simulink model "tutorial36_stateflow"  (R2025a)
settings: Solver=VariableStepAuto  StartTime=0.0  StopTime=10.0  RelTol=1e-3
settings Model: Creator=xing2  LastModifiedBy=xing2

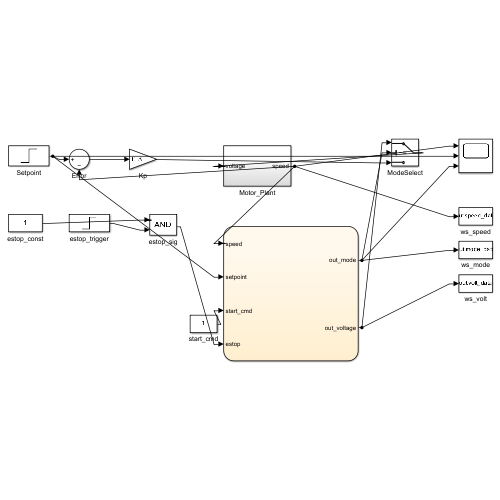
[thumbnail: Simulink's stored preview of the top-level diagram]
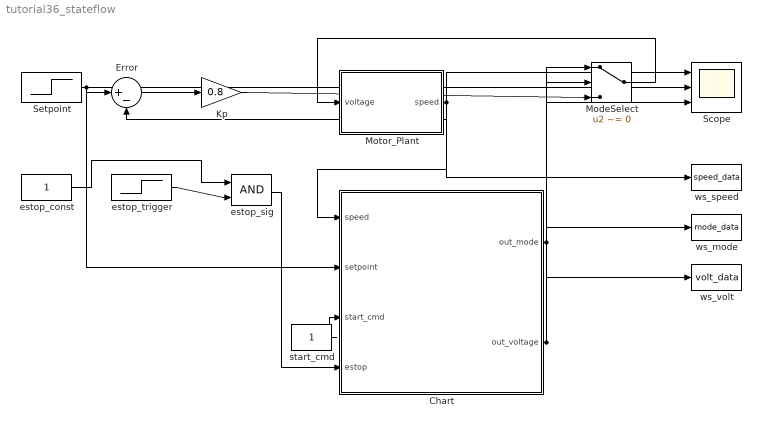
== system tutorial36_stateflow ==
  Chart : Stateflow chart  TreatAsAtomicUnit=on
  Error : Sum  Inputs=|+-
  Kp : Gain  Gain=0.8
  ModeSelect : Switch  Criteria=u2 ~= 0  SaturateOnIntegerOverflow=off  InputSameDT=off
  Motor_Plant : Subsystem
  Scope : Scope  NumInputPorts=3
  Setpoint : Step  Time=0.5  After=100  SampleTime=0
  estop_const : Constant
  estop_sig : Logic  AllPortsSameDT=off  OutDataTypeStr=boolean
  estop_trigger : Step  Time=8  SampleTime=0
  start_cmd : Constant
  ws_mode : ToWorkspace  VariableName=mode_data  SaveFormat=Timeseries  SampleTime=-1
  ws_speed : ToWorkspace  VariableName=speed_data  SaveFormat=Timeseries  SampleTime=-1
  ws_volt : ToWorkspace  VariableName=volt_data  SaveFormat=Timeseries  SampleTime=-1
  wires:
  Motor_Plant/1(speed) -> Chart/1(speed), Error/2, Scope/1, ws_speed/1
  Setpoint/1 -> Chart/2(setpoint), Error/1, Scope/2
  start_cmd/1 -> Chart/3(start_cmd)
  estop_const/1 -> estop_sig/1
  estop_trigger/1 -> estop_sig/2
  estop_sig/1 -> Chart/4(estop)
  Error/1 -> Kp/1
  Kp/1 -> ModeSelect/3
  Chart/2(out_voltage) -> ModeSelect/1, ws_volt/1
  Chart/1(out_mode) -> ModeSelect/2, Scope/3, ws_mode/1
  ModeSelect/1 -> Motor_Plant/1(voltage)

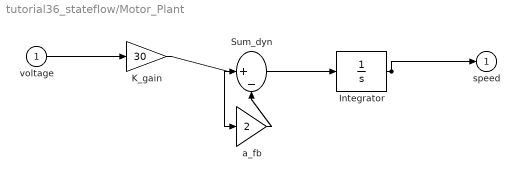
== system tutorial36_stateflow/Motor_Plant ==
  voltage : Inport
  Integrator : Integrator
  K_gain : Gain  Gain=30
  Sum_dyn : Sum  Inputs=|+-
  a_fb : Gain  Gain=2
  speed : Outport
  wires:
  voltage/1 -> K_gain/1
  K_gain/1 -> Sum_dyn/1
  Sum_dyn/1 -> Integrator/1
  Integrator/1 -> a_fb/1, speed/1
  a_fb/1 -> Sum_dyn/2

== stateflow chart tutorial36_stateflow/Chart ==
  state STARTING
    en: out_mode = 1;
    du: out_voltage = min(10, out_voltage + 0.2);
  state OFF
    en: out_mode = 0;
    out_voltage = 0;
  state RUNNING
    en: out_mode = 2;
    out_voltage = Kp*(setpoint - speed);
  (default) -> OFF
  STARTING -> OFF [order 2] : [estop == 1]
  RUNNING -> OFF : [estop == 1]
  OFF -> STARTING : [start_cmd == 1]
  STARTING -> RUNNING [order 1] : [speed >= 80]
  data: speed input; setpoint input; start_cmd input; estop input; out_mode output; out_voltage output; Kp constant double =0.8
